simulink model "lab_01_simulink_lazo_abierto"  (R2016a)
settings: Solver=FixedStepAuto  StartTime=0.0  StopTime=10.0  RelTol=1e-3
undefined symbols (not defined in the file): serial
libraries: instrumentlib x3
settings Model: Creator=dcasta25  LastModifiedBy=dcasta25

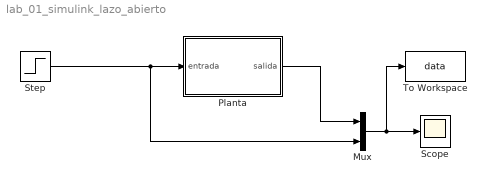
== system lab_01_simulink_lazo_abierto ==
  Mux : Mux  Inputs=2
  Planta : Subsystem
  Scope : Scope
  Step : Step  Time=3  After=200  SampleTime=0.1
  To Workspace : ToWorkspace  VariableName=data  SaveFormat=Timeseries  SampleTime=-1
  wires:
  Step/1 -> Mux/2, Planta/1(entrada)
  Planta/1(salida) -> Mux/1
  Mux/1 -> To Workspace/1, Scope/1

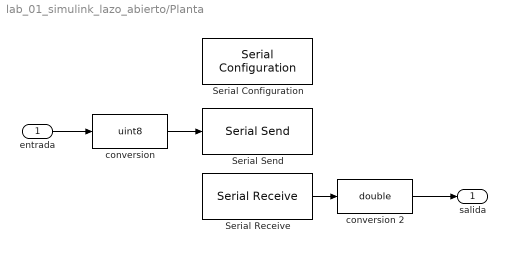
== system lab_01_simulink_lazo_abierto/Planta ==
  entrada : Inport
  Serial Configuration : instrumentlib/Serial Configuration  Priority=-200000  ComPortMenu=COM7  ComPort=COM7  ObjConstructor=serial('COM7');  BaudRate=9600  DataBits=8  Parity=none  StopBits=1  FlowControl=none  Timeout=10  ByteOrder=LittleEndian
  Serial Receive : instrumentlib/Serial Receive  ComPortMenu=COM7  ComPort=COM7  ObjConstructor=serial('COM7');  Terminator=<none>  DataSize=[1 1]  DataType=uint8  EnableBlockingMode=on  ActionDataUnavailable=Output last received value  CustomValue=0  SampleTime=0.1
  Serial Send : instrumentlib/Serial Send  ComPortMenu=COM7  ComPort=COM7  ObjConstructor=serial('COM7');  Terminator=<none>  EnableBlockingMode=on
  conversion : DataTypeConversion  OutDataTypeStr=uint8
  conversion 2 : DataTypeConversion  OutDataTypeStr=double
  salida : Outport
  wires:
  entrada/1 -> conversion/1
  conversion 2/1 -> salida/1
  Serial Receive/1 -> conversion 2/1
  conversion/1 -> Serial Send/1
